simulink model "sintonizar1d6"  (Simulink 2.09)
settings: Solver=ode45  StartTime=0.0  StopTime=0.5  MaxStep=0.1  RelTol=1e-3  AbsTol=1e-3
settings Model: SaveTime=off  SaveOutput=off  ConsistencyChecking=off  RTWTemplateMakefile=grt_vc.tmf

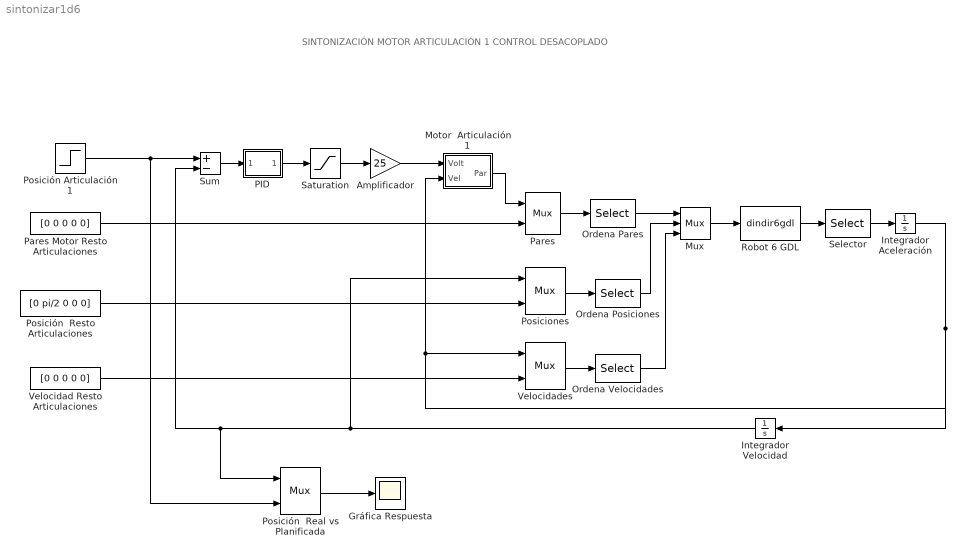
== system sintonizar1d6 ==
  note: SINTONIZACIÓN MOTOR ARTICULACIÓN 1
      | CONTROL DESACOPLADO
  Amplificador : Gain  Gain=25
  Gráfica Respuesta : Scope
      settings: TickLabels=on  TimeRange=auto  YMin=-8.67362e-018  YMax=0.08500000000000001  SaveToWorkspace=off  SaveName=ScopeData  LimitMaxRows=off  MaxRows=500
  Integrador Aceleración : Integrator  ExternalReset=none  InitialConditionSource=internal  InitialCondition=0  LimitOutput=off  UpperSaturationLimit=inf  LowerSaturationLimit=-inf  ShowSaturationPort=off  ShowStatePort=off  AbsoluteTolerance=auto
  Integrador Velocidad : Integrator  Orientation=left  ExternalReset=none  InitialConditionSource=internal  InitialCondition=0  LimitOutput=off  UpperSaturationLimit=inf  LowerSaturationLimit=-inf  ShowSaturationPort=off  ShowStatePort=off  AbsoluteTolerance=auto
  Motor  Articulación 1 : Subsystem  mask(Motor){R=0.8, L=0.00093, Kt=0.058, Kv=0.058, imax=18.5, red=500}
      mask prompts: R "Resistencia (Ohmios)"; L "Inductancia (Henrios)"; Kt "Kt (Nm/A)"; Kv "Kv (V/rad/s)"; imax "Corriente máxima (Amperios)"; red "Reductor"
  Mux : Mux  Inputs=3
  Ordena Pares : Selector  Elements=[1 2 3 4 5 6]  InputPortWidth=6
  Ordena Posiciones : Selector  Elements=[1 2 3 4 5 6]  InputPortWidth=6
  Ordena Velocidades : Selector  Elements=[1 2 3 4 5 6]  InputPortWidth=6
  PID : Subsystem  mask(PID Controller){P=500, I=0, D=12}
      mask prompts: P "Proportional:"; I "Integral"; D "Derivative:"
      mask help:
      | Enter expressions for proportional, integral, and derivative terms.
      | P+I/s+Ds
      mask Help: This block implements a PID controller where parameters are entered for the Proportional, Integral and Derivative terms. Unmask this block to see how it works. The derivative term is implemented using a true derivative block.
      mask Display: disp('PID')
  Pares : Mux  Inputs=2
  Pares Motor Resto Articulaciones : Constant  Value=[0 0 0 0 0]
  Posiciones : Mux  Inputs=2
  Posición Articulación 1 : Step  Time=0  Before=0  After=0.08
  Posición  Real vs Planificada : Mux  Inputs=2
  Posición  Resto Articulaciones : Constant  Value=[0 pi/2 0 0 0]
  Robot 6 GDL : MATLABFcn  MATLABFcn=dindir6gdl  OutputWidth=6
  Saturation : Saturate  UpperLimit=10  LowerLimit=-10
  Selector : Selector  Elements=1  InputPortWidth=6
  Sum : Sum  Inputs=+-
  Velocidad Resto Articulaciones : Constant  Value=[0 0 0 0 0]
  Velocidades : Mux  Inputs=2
  wires:
  Pares Motor Resto Articulaciones/1 -> Pares/2
  Saturation/1 -> Amplificador/1
  PID/1(Out_1) -> Saturation/1
  Sum/1 -> PID/1(In_1)
  Mux/1 -> Robot 6 GDL/1
  Amplificador/1 -> Motor  Articulación 1/1(Volt)
  Motor  Articulación 1/1(Par) -> Pares/1
  Posición  Resto Articulaciones/1 -> Posiciones/2
  Integrador Velocidad/1 -> Posiciones/1, Sum/2, Posición  Real vs Planificada/1
  Velocidad Resto Articulaciones/1 -> Velocidades/2
  Posición Articulación 1/1 -> Sum/1, Posición  Real vs Planificada/2
  Robot 6 GDL/1 -> Selector/1
  Posición  Real vs Planificada/1 -> Gráfica Respuesta/1
  Selector/1 -> Integrador Aceleración/1
  Integrador Aceleración/1 -> Integrador Velocidad/1, Motor  Articulación 1/2(Vel), Velocidades/1
  Pares/1 -> Ordena Pares/1
  Ordena Pares/1 -> Mux/1
  Posiciones/1 -> Ordena Posiciones/1
  Ordena Posiciones/1 -> Mux/2
  Velocidades/1 -> Ordena Velocidades/1
  Ordena Velocidades/1 -> Mux/3

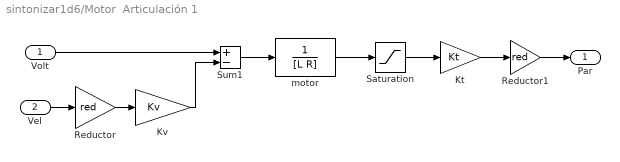
== system sintonizar1d6/Motor  Articulación 1 ==
  Volt : Inport  Port=1  PortWidth=-1  SampleTime=-1
  Vel : Inport  Port=2  PortWidth=-1  SampleTime=-1
  Kt : Gain  Gain=Kt
  Kv : Gain  Gain=Kv
  Reductor : Gain  Gain=red
  Reductor1 : Gain  Gain=red
  Saturation : Saturate  UpperLimit=imax  LowerLimit=-imax
  Sum1 : Sum  Inputs=+-
  motor : TransferFcn  Numerator=[1]  Denominator=[L R]
  Par : Outport  Port=1  InitialOutput=0
  wires:
  Vel/1 -> Reductor/1
  Volt/1 -> Sum1/1
  Kv/1 -> Sum1/2
  Reductor/1 -> Kv/1
  Sum1/1 -> motor/1
  Reductor1/1 -> Par/1
  Kt/1 -> Reductor1/1
  motor/1 -> Saturation/1
  Saturation/1 -> Kt/1

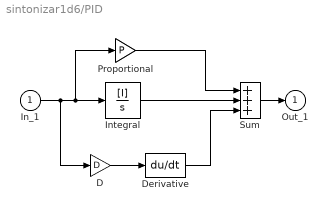
== system sintonizar1d6/PID ==
  In_1 : Inport  Port=1  PortWidth=-1  SampleTime=-1
  D : Gain  Gain=D
  Derivative : Derivative
  Integral : TransferFcn  Numerator=[I]  Denominator=[1 0]
  Proportional : Gain  Gain=P
  Sum : Sum  Inputs=+++
  Out_1 : Outport  Port=1  InitialOutput=0
  wires:
  D/1 -> Derivative/1
  Sum/1 -> Out_1/1
  In_1/1 -> D/1, Integral/1, Proportional/1
  Derivative/1 -> Sum/3
  Integral/1 -> Sum/2
  Proportional/1 -> Sum/1
